simulink model "HLB_trp_test"  (R2019b)
settings: Solver=FixedStepDiscrete  StartTime=0.0  StopTime=1000.0  FixedStep=0.05  RelTol=1e-3
settings Model: Creator=DOT1BP  LastModifiedBy=DOT1BP

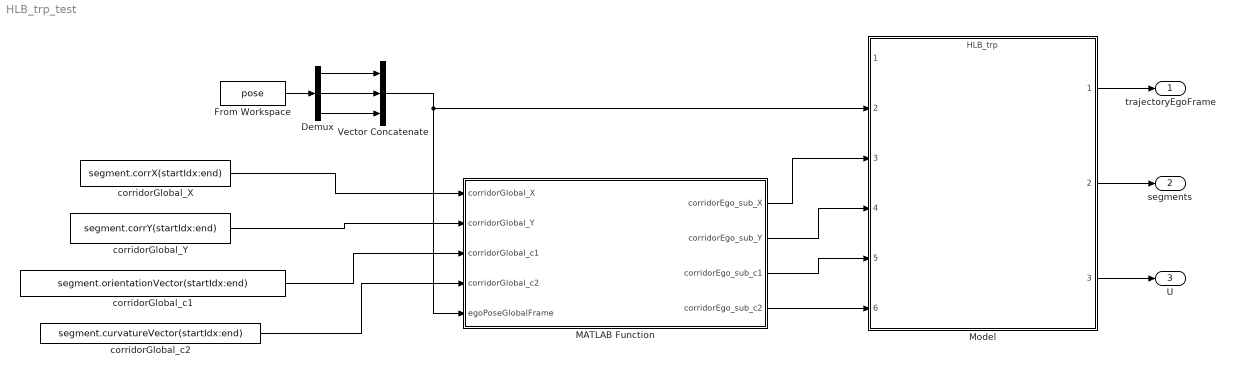
== system HLB_trp_test ==
  Demux : Demux  Outputs=3
  From Workspace : FromWorkspace  VariableName=pose
  MATLAB Function : MATLAB Function  TreatAsAtomicUnit=on
  Model : ModelReference  ModelNameDialog=HLB_trp.slx  SimulationMode=Normal  ModelReferenceVersion=1.896
  Vector Concatenate : Concatenate  NumInputs=3
  corridorGlobal_X : Constant  Value=segment.corrX(startIdx:end)
  corridorGlobal_Y : Constant  Value=segment.corrY(startIdx:end)
  corridorGlobal_c1 : Constant  Value=segment.orientationVector(startIdx:end)
  corridorGlobal_c2 : Constant  Value=segment.curvatureVector(startIdx:end)
  trajectoryEgoFrame : Outport
  segments : Outport  Port=2
  U : Outport  Port=3
  wires:
  corridorGlobal_c1/1 -> MATLAB Function/3(corridorGlobal_c1)
  Vector Concatenate/1 -> Model/2, MATLAB Function/5(egoPoseGlobalFrame)
  From Workspace/1 -> Demux/1
  Demux/1 -> Vector Concatenate/1
  corridorGlobal_Y/1 -> MATLAB Function/2(corridorGlobal_Y)
  Demux/3 -> Vector Concatenate/3
  corridorGlobal_X/1 -> MATLAB Function/1(corridorGlobal_X)
  Demux/2 -> Vector Concatenate/2
  corridorGlobal_c2/1 -> MATLAB Function/4(corridorGlobal_c2)
  MATLAB Function/4(corridorEgo_sub_c2) -> Model/6
  MATLAB Function/3(corridorEgo_sub_c1) -> Model/5
  MATLAB Function/2(corridorEgo_sub_Y) -> Model/4
  MATLAB Function/1(corridorEgo_sub_X) -> Model/3
  Model/1 -> trajectoryEgoFrame/1
  Model/2 -> segments/1
  Model/3 -> U/1

== matlab function HLB_trp_test/MATLAB Function ==
  data: corridorGlobal_X input; corridorEgo_sub_X output; corridorGlobal_Y input; corridorGlobal_c1 input; corridorGlobal_c2 input; egoPoseGlobalFrame input; corridorEgo_sub_Y output; corridorEgo_sub_c1 output; corridorEgo_sub_c2 output
function [corridorEgo_sub_X, corridorEgo_sub_Y, corridorEgo_sub_c1, corridorEgo_sub_c2] = subsegment_cutting(corridorGlobal_X, corridorGlobal_Y, corridorGlobal_c1, corridorGlobal_c2, egoPoseGlobalFrame)

corridorGlobal_sub_X = zeros(301,1);
corridorGlobal_sub_Y = zeros(301,1);
corridorGlobal_sub_c1 = zeros(301,1);
corridorGlobal_sub_c2 = zeros(301,1);

corridorEgo_sub_X = zeros(301,1);
corridorEgo_sub_Y = zeros(301,1);
corridorEgo_sub_c1 = zeros(301,1);
corridorEgo_sub_c2 = zeros(301,1);

corridorEgo = zeros(300,2);

distances_vec = ((corridorGlobal_X - egoPoseGlobalFrame(1)).^2 + (corridorGlobal_Y - egoPoseGlobalFrame(2)).^2).^0.5;

[closest_point_index] = find(distances_vec == min(distances_vec),1);
[closest_toLAD_index] = find(distances_vec(closest_point_index(1):end) > 150, 1);
closest_point_index = closest_point_index(1);
closest_toLAD_index = closest_toLAD_index(1);

n = closest_point_index + closest_toLAD_index;

corridorGlobal_sub_X(1:closest_toLAD_index+1,1) = corridorGlobal_X(closest_point_index:n,1);
corridorGlobal_sub_Y(1:closest_toLAD_index+1,1) = corridorGlobal_Y(closest_point_index:n,1);
corridorGlobal_sub_c1(1:closest_toLAD_index+1,1) = corridorGlobal_c1(closest_point_index:n,1);
corridorGlobal_sub_c2(1:closest_toLAD_index+1,1) = corridorGlobal_c2(closest_point_index:n,1);

T = [cos(egoPoseGlobalFrame(3)) sin(egoPoseGlobalFrame(3)); -sin(egoPoseGlobalFrame(3)) cos(egoPoseGlobalFrame(3))];
corridorEgo(1:closest_toLAD_index+1,1:2) = [corridorGlobal_sub_X(1:closest_toLAD_index+1,1)-egoPoseGlobalFrame(1) corridorGlobal_sub_Y(1:closest_toLAD_index+1,1)-egoPoseGlobalFrame(2)]*T';

corridorEgo_sub_X(1:closest_toLAD_index+1,1) = corridorEgo(1:closest_toLAD_index+1,1);
corridorEgo_sub_Y(1:closest_toLAD_index+1,1) = corridorEgo(1:closest_toLAD_index+1,2);
corridorEgo_sub_c1(1:closest_toLAD_index+1,1) = corridorGlobal_sub_c1(1:closest_toLAD_index+1,1) - egoPoseGlobalFrame(3);
corridorEgo_sub_c2(1:closest_toLAD_index+1,1) = corridorGlobal_sub_c2(1:closest_toLAD_index+1,1);

corridorEgo_sub_X(301) = closest_toLAD_index+1;
corridorEgo_sub_Y(301) = closest_toLAD_index+1;
corridorEgo_sub_c1(301) = closest_toLAD_index+1;
corridorEgo_sub_c2(301) = closest_toLAD_index+1;


end
